simulink library "sn3218"  (R2026a)
settings: Solver=VariableStepAuto
libraries: raspberrypiCommlib x5
settings Model: Creator=ebene  LastModifiedBy=ebene

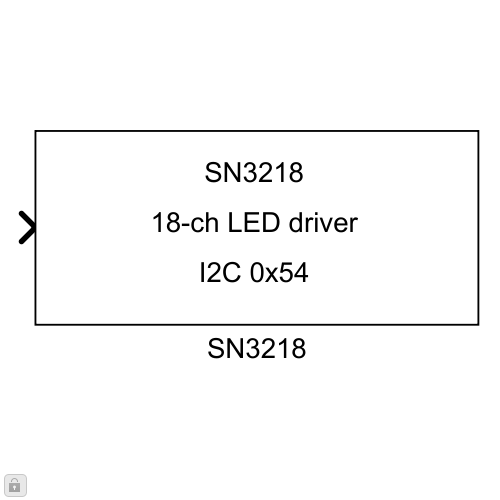
[thumbnail: Simulink's stored preview of the top-level diagram]
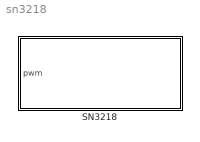
== system sn3218 ==
  SN3218 : Subsystem  mask(SN3218){Board=Pi 3 Model B+}
      mask prompts: Board "Hardware board:"
      mask help:
      | SN3218 18-channel I2C LED driver (address 0x54).
      |
      | pwm: uint8 [18x1] per-channel brightness, mapped to registers 0x01-0x12.
      |
      | At initialisation an Initialize Function subsystem resets the device
      | (0x17), enables normal operation (0x00) and turns on all 18 output
      | enables (0x13-0x15). Every step thereafter it gamma-corrects pwm, writes
      | the 18 PWM registers and latches them via the update register (0x16).
      |
      | Gamma is a 2.2 power law, which preserves both endpoints: 0 is fully off
      | and 255 is fully on. Comment-through the Gamma block to drive the device
      | with uncorrected values.
      |
      | No GPIO is driven: the SN3218 SDB pin is tied active on Trilobot, and
      | enable/disable is the 0x00 shutdown register over I2C.
      |
      | Board sets the hardware board on every inner I2C block. The I2C bus (1)
      | is still set on the inner blocks.
      mask init:
      | targets = {'Init/Reset 0x17', 'Init/Shutdown 0x00', ...
      |     'Init/LED Enable 0x13', 'PWM 0x01', 'Update 0x16'};
      | for i = 1:numel(targets)
      |     blk = [gcb '/' targets{i}];
      |     if ~strcmp(get_param(blk, 'BoardProperty'), Board)
      |         set_param(blk, 'BoardProperty', Board);
      |     end
      | end
      mask TypeOptions Board: Model B Rev1 | Model B Rev2 | Model B+ | Pi 2 Model B | Pi 3 Model B | Pi 3 Model B+ | Pi Zero W | Pi 4 Model B | Compute Module 4 | Pi Zero 2 W | Pi 5 Model | Compute Module 5
      mask Display:
      | color('black');
      | text(0.5, 0.80, 'SN3218', 'horizontalAlignment', 'center');
      | text(0.5, 0.55, '18-ch LED driver', 'horizontalAlignment', 'center');
      | text(0.5, 0.28, 'I2C 0x54', 'horizontalAlignment', 'center');

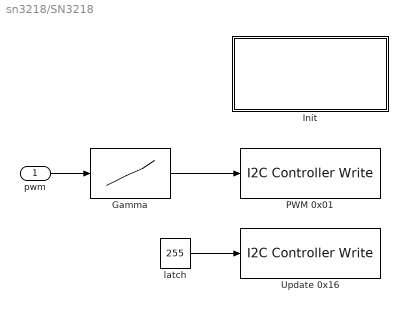
== system sn3218/SN3218 ==
  pwm : Inport  OutDataTypeStr=uint8  PortDimensions=18
  Gamma : Lookup_n-D  NumberOfTableDimensions=1  BreakpointsForDimension1=0:255  Table=uint8(round(255*((0:255)/255).^2.2))  ExtrapMethod=Clip  InternalRulePriority=Speed  OutDataTypeStr=uint8  RndMeth=Simplest
  Init : Subsystem  TreatAsAtomicUnit=on
  PWM 0x01 : raspberrypiCommlib/I2C Controller Write  Priority=2  BoardProperty=Pi 3 Model B+  I2CModule=1  Mode=Master  SlaveAddress=84  SlaveByteOrder=BigEndian  Direction=Transmitter  RegisterAddressMode=on  RegisterAddress=1  SlaveDataType=uint8  DataLength=1  NoAck=off  RepeatedStart=off  OutputStatus=off
  Update 0x16 : raspberrypiCommlib/I2C Controller Write  Priority=3  BoardProperty=Pi 3 Model B+  I2CModule=1  Mode=Master  SlaveAddress=84  SlaveByteOrder=BigEndian  Direction=Transmitter  RegisterAddressMode=on  RegisterAddress=22  SlaveDataType=uint8  DataLength=1  NoAck=off  RepeatedStart=off  OutputStatus=off
  latch : Constant  Value=255  OutDataTypeStr=uint8
  wires:
  pwm/1 -> Gamma/1
  Gamma/1 -> PWM 0x01/1
  latch/1 -> Update 0x16/1

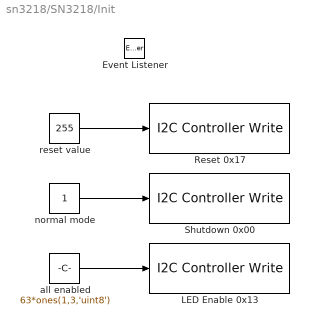
== system sn3218/SN3218/Init ==
  Event Listener : EventListener  DisableCoverage=on  EventName=reset
  LED Enable 0x13 : raspberrypiCommlib/I2C Controller Write  Priority=3  BoardProperty=Pi 3 Model B+  I2CModule=1  Mode=Master  SlaveAddress=84  SlaveByteOrder=BigEndian  Direction=Transmitter  RegisterAddressMode=on  RegisterAddress=19  SlaveDataType=uint8  DataLength=1  NoAck=off  RepeatedStart=off  OutputStatus=off
  Reset 0x17 : raspberrypiCommlib/I2C Controller Write  Priority=1  BoardProperty=Pi 3 Model B+  I2CModule=1  Mode=Master  SlaveAddress=84  SlaveByteOrder=BigEndian  Direction=Transmitter  RegisterAddressMode=on  RegisterAddress=23  SlaveDataType=uint8  DataLength=1  NoAck=off  RepeatedStart=off  OutputStatus=off
  Shutdown 0x00 : raspberrypiCommlib/I2C Controller Write  Priority=2  BoardProperty=Pi 3 Model B+  I2CModule=1  Mode=Master  SlaveAddress=84  SlaveByteOrder=BigEndian  Direction=Transmitter  RegisterAddressMode=on  RegisterAddress=0  SlaveDataType=uint8  DataLength=1  NoAck=off  RepeatedStart=off  OutputStatus=off
  all enabled : Constant  Value=63*ones(1,3,'uint8')  OutDataTypeStr=uint8
  normal mode : Constant  OutDataTypeStr=uint8
  reset value : Constant  Value=255  OutDataTypeStr=uint8
  wires:
  reset value/1 -> Reset 0x17/1
  all enabled/1 -> LED Enable 0x13/1
  normal mode/1 -> Shutdown 0x00/1
